simulink model "Expt2_19EE30012_ModiOmkar_QuesA"  (R2020b)
settings: Solver=VariableStepAuto  StartTime=0.0  StopTime=0.001  MaxStep=1e-7  RelTol=1e-3
libraries: powerlib x12, eeGeneralControl x1, powerlib_meascontrol x1
settings Model: Creator=win10  LastModifiedBy=HP

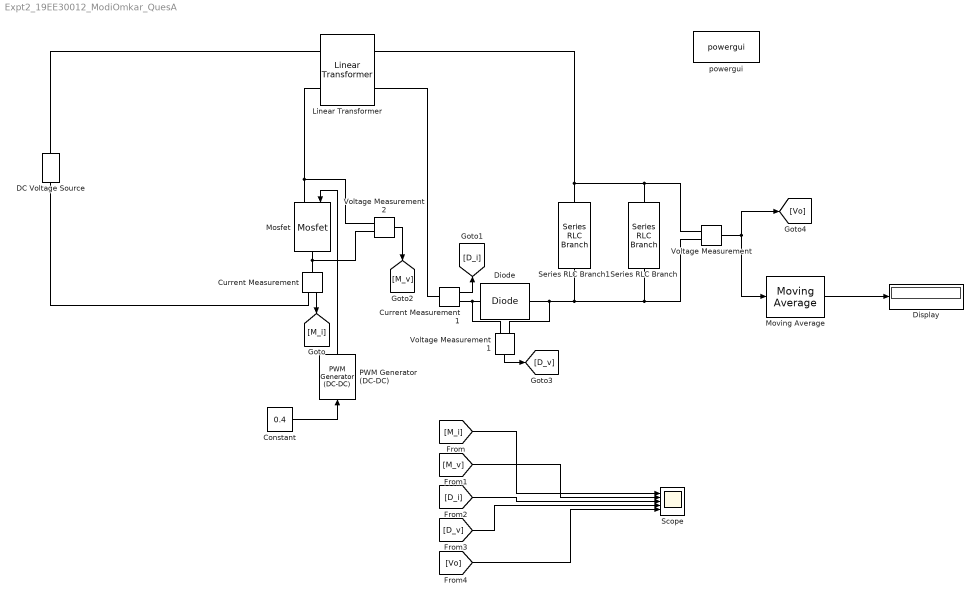
== system Expt2_19EE30012_ModiOmkar_QuesA ==
  Constant : Constant  Value=0.4
  Current Measurement : powerlib/Measurements/Current Measurement  PhasorSimulation=off  OutputType=Complex  PSBequivalent=0
  Current Measurement1 : powerlib/Measurements/Current Measurement  PhasorSimulation=off  OutputType=Complex  PSBequivalent=0
  DC Voltage Source : powerlib/Electrical Sources/DC Voltage Source  Amplitude=20  Measurements=None
  Diode : powerlib/Power Electronics/Diode  Ron=1e-6  Lon=0  Vf=0  IC=0  UseSnubber=0  Rs=1e12  Cs=0  Measurements=off
  Display : Display
      settings: Format=bank
  Linear Transformer : powerlib/Elements/Linear Transformer  UNITS=SI  NominalPower=[100 100e3]  winding1=[20 0 0]  winding2=[4 0 0]  ThreeWindings=off  winding3=[3.15e+05 1.9845e+06 2.5267e+05]  RmLm=[1e12 20e-6]  Measurements=None  DataType=on
  Mosfet : powerlib/Power Electronics/Mosfet  Ron=1e-6  Lon=0  Rd=1e-6  Vfd=0  IC=0  Rs=1e12  Cs=inf  Measurements=off
  Moving Average : eeGeneralControl/Moving Average  VariantControl=Variant1  LabelModeActiveChoice=Discrete  f=100e3  x0=0  Ts=-1
      settings: SourceProductBaseCode=PS
  PWM Generator (DC-DC) : powerlib_meascontrol/Pulse & Signal Generators/PWM Generator (DC-DC)  Fsw=100e3  Ts=0
  Scope : Scope  NumInputPorts=5
  Series RLC Branch : powerlib/Elements/Series RLC Branch  LConnTagsString=__new0  RConnTagsString=__new0  BranchType=R  Resistance=1  Inductance=1e-3  SetiL0=off  InitialCurrent=0  Capacitance=1e-6  Setx0=off  InitialVoltage=0  Measurements=None
  Series RLC Branch1 : powerlib/Elements/Series RLC Branch  LConnTagsString=__new0  RConnTagsString=__new0  BranchType=C  Resistance=1  Inductance=1e-3  SetiL0=off  InitialCurrent=0  Capacitance=100e-6  Setx0=off  InitialVoltage=0  Measurements=None
  Voltage Measurement : powerlib/Measurements/Voltage Measurement  PhasorSimulation=off  OutputType=Complex  PSBequivalent=0
  Voltage Measurement1 : powerlib/Measurements/Voltage Measurement  PhasorSimulation=off  OutputType=Complex  PSBequivalent=0
  Voltage Measurement2 : powerlib/Measurements/Voltage Measurement  PhasorSimulation=off  OutputType=Complex  PSBequivalent=0
  powergui : powerlib/powergui  Priority=1  SimulationMode=Discrete  SampleTime=1e-7  frequency=60  Iterations=50  frequencyindice=0  Pbase=100e6  ErrMax=1e-4  UnitsV=kV  UnitsW=MW  buscounter=0  FunctionMessages=off  echomessages=off  EnableUseOfTLC=off  CurrentSourceSwitches=off  DisableSnubberDevices=off  DisableRonSwitches=off  DisableVfSwitches=off  DisplayEquations=off  AutomaticDiscreteSolvers=off  SolverType=Tustin/Backward Euler (TBE)  Interpol=off  ExternalGateDelay=off  methode=off  Ts=100  x0status=blocks  SPID=on  SwTol=0  HookPort=off  NonlinearTolerance=1e-4  nMaxIteration=100  ContinueOnMaxIteration=off  RestoreLinks=warning  ResistiveCurrentMeasurement=off  Frange=[0:2:500]  Ylog=off  Xlog=on  ShowGrid=off  save=off  variable=ZData  structure=0  ZoomFFT=off  StartTime=0.0  cycles=1  DisplayStyle=1  fundamental=60  FreqAxis=off  MaxFrequency=1000  frequencyindicesteady=1  RmsSteady=1  display=off
  wires:
  PWM Generator (DC-DC)/1 -> Mosfet/1
  Voltage Measurement/1 -> [Vo], Moving Average/1
  Moving Average/1 -> Display/1
  Constant/1 -> PWM Generator (DC-DC)/1
  Current Measurement/1 -> [M_i]
  Voltage Measurement2/1 -> [M_v]
  Current Measurement1/1 -> [D_i]
  Voltage Measurement1/1 -> [D_v]
  [M_i] -> Scope/1
  [M_v] -> Scope/2
  [D_i] -> Scope/3
  [D_v] -> Scope/4
  [Vo] -> Scope/5
  connections:
  Mosfet/LConn1 -- Linear Transformer/LConn2 -- Voltage Measurement2/LConn1
  Diode/RConn1 -- Voltage Measurement/LConn2 -- Series RLC Branch/LConn1 -- Series RLC Branch1/LConn1 -- Voltage Measurement1/LConn2
  Series RLC Branch/RConn1 -- Voltage Measurement/LConn1 -- Linear Transformer/RConn1 -- Series RLC Branch1/RConn1
  DC Voltage Source/RConn1 -- Linear Transformer/LConn1
  Current Measurement/LConn1 -- Voltage Measurement2/LConn2 -- Mosfet/RConn1
  Current Measurement/RConn1 -- DC Voltage Source/LConn1
  Diode/LConn1 -- Voltage Measurement1/LConn1 -- Current Measurement1/RConn1
  Linear Transformer/RConn2 -- Current Measurement1/LConn1
